simulink model "twsbr_fuzzy_pid"  (R2026a)
settings: Solver=ode45  StopTime=8.0  MaxStep=0.001  RelTol=1e-9  AbsTol=1e-11
model workspace (MAT data in the model file):
  controller_reset_data = [0  1; 0.001  0; 8  0]
  disturbance_force_data = [0  0; 8  0]
  disturbance_torque_data = [0  0; 8  0]
  position_reference_data = [0  0; 8  0]
settings Model: Creator=Linxiuqi  LastModifiedBy=Linxiuqi

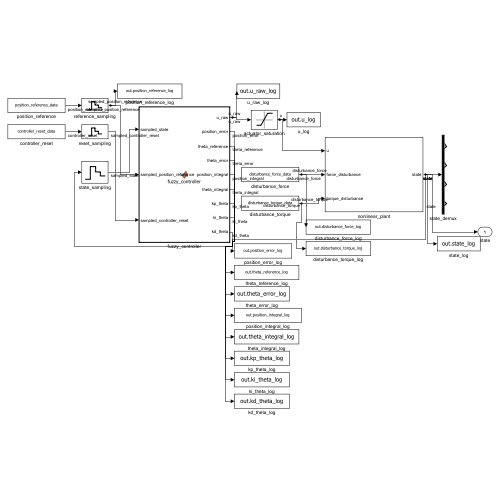
[thumbnail: Simulink's stored preview of the top-level diagram]
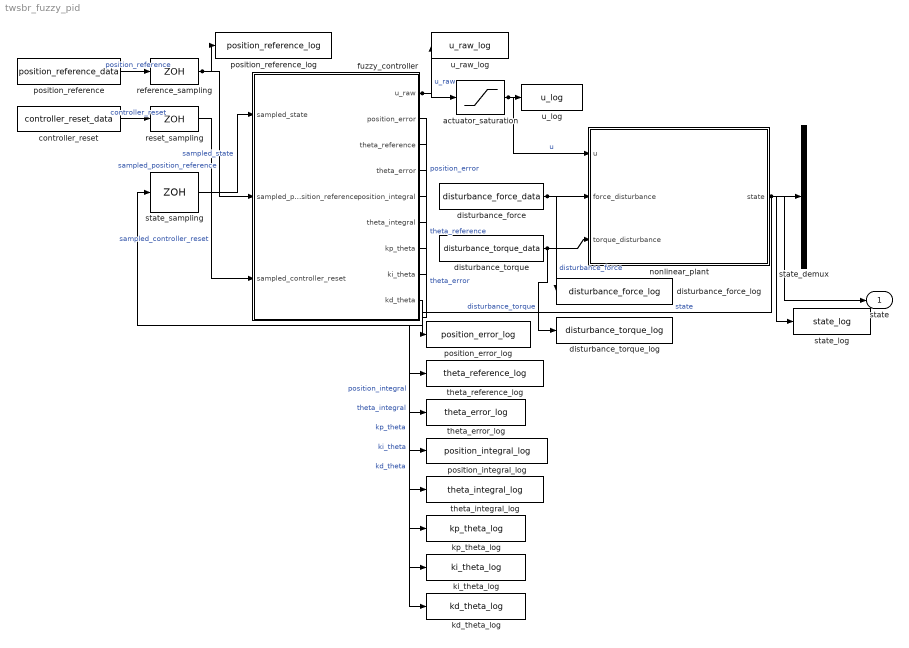
== system twsbr_fuzzy_pid ==
  actuator_saturation : Saturate  UpperLimit=1  LowerLimit=-1
  controller_reset : FromWorkspace  VariableName=controller_reset_data  Interpolate=off  OutputAfterFinalValue=Holding final value
  disturbance_force : FromWorkspace  VariableName=disturbance_force_data  Interpolate=off  OutputAfterFinalValue=Holding final value
  disturbance_force_log : ToWorkspace  VariableName=disturbance_force_log  SaveFormat=Structure With Time  SampleTime=-1
  disturbance_torque : FromWorkspace  VariableName=disturbance_torque_data  Interpolate=off  OutputAfterFinalValue=Holding final value
  disturbance_torque_log : ToWorkspace  VariableName=disturbance_torque_log  SaveFormat=Structure With Time  SampleTime=-1
  fuzzy_controller : MATLAB Function  TreatAsAtomicUnit=on
  kd_theta_log : ToWorkspace  VariableName=kd_theta_log  SaveFormat=Structure With Time  SampleTime=-1
  ki_theta_log : ToWorkspace  VariableName=ki_theta_log  SaveFormat=Structure With Time  SampleTime=-1
  kp_theta_log : ToWorkspace  VariableName=kp_theta_log  SaveFormat=Structure With Time  SampleTime=-1
  nonlinear_plant : Subsystem
  position_error_log : ToWorkspace  VariableName=position_error_log  SaveFormat=Structure With Time  SampleTime=-1
  position_integral_log : ToWorkspace  VariableName=position_integral_log  SaveFormat=Structure With Time  SampleTime=-1
  position_reference : FromWorkspace  VariableName=position_reference_data  Interpolate=off  OutputAfterFinalValue=Holding final value
  position_reference_log : ToWorkspace  VariableName=position_reference_log  SaveFormat=Structure With Time  SampleTime=-1
  reference_sampling : ZeroOrderHold  SampleTime=0.01
  reset_sampling : ZeroOrderHold  SampleTime=0.01
  state_demux : Demux
  state_log : ToWorkspace  VariableName=state_log  SaveFormat=Structure With Time  SampleTime=-1
  state_sampling : ZeroOrderHold  SampleTime=0.01
  theta_error_log : ToWorkspace  VariableName=theta_error_log  SaveFormat=Structure With Time  SampleTime=-1
  theta_integral_log : ToWorkspace  VariableName=theta_integral_log  SaveFormat=Structure With Time  SampleTime=-1
  theta_reference_log : ToWorkspace  VariableName=theta_reference_log  SaveFormat=Structure With Time  SampleTime=-1
  u_log : ToWorkspace  VariableName=u_log  SaveFormat=Structure With Time  SampleTime=-1
  u_raw_log : ToWorkspace  VariableName=u_raw_log  SaveFormat=Structure With Time  SampleTime=-1
  state : Outport
  wires:
  position_reference/1 -> reference_sampling/1  "position_reference"
  reference_sampling/1 -> fuzzy_controller/2(sampled_position_reference), position_reference_log/1  "sampled_position_reference"
  controller_reset/1 -> reset_sampling/1  "controller_reset"
  reset_sampling/1 -> fuzzy_controller/3(sampled_controller_reset)  "sampled_controller_reset"
  nonlinear_plant/1(state) -> state_sampling/1, state_demux/1, state/1, state_log/1  "state"
  state_sampling/1 -> fuzzy_controller/1(sampled_state)  "sampled_state"
  fuzzy_controller/1(u_raw) -> actuator_saturation/1, u_raw_log/1  "u_raw"
  fuzzy_controller/2(position_error) -> position_error_log/1  "position_error"
  fuzzy_controller/3(theta_reference) -> theta_reference_log/1  "theta_reference"
  fuzzy_controller/4(theta_error) -> theta_error_log/1  "theta_error"
  fuzzy_controller/5(position_integral) -> position_integral_log/1  "position_integral"
  fuzzy_controller/6(theta_integral) -> theta_integral_log/1  "theta_integral"
  fuzzy_controller/7(kp_theta) -> kp_theta_log/1  "kp_theta"
  fuzzy_controller/8(ki_theta) -> ki_theta_log/1  "ki_theta"
  fuzzy_controller/9(kd_theta) -> kd_theta_log/1  "kd_theta"
  actuator_saturation/1 -> nonlinear_plant/1(u), u_log/1  "u"
  disturbance_force/1 -> nonlinear_plant/2(force_disturbance), disturbance_force_log/1  "disturbance_force"
  disturbance_torque/1 -> nonlinear_plant/3(torque_disturbance), disturbance_torque_log/1  "disturbance_torque"

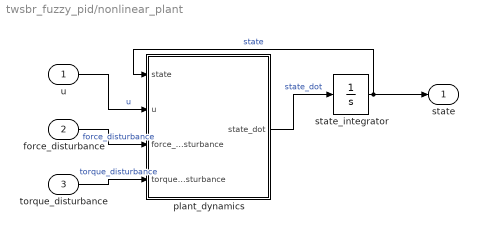
== system twsbr_fuzzy_pid/nonlinear_plant ==
  u : Inport
  force_disturbance : Inport  Port=2
  torque_disturbance : Inport  Port=3
  plant_dynamics : MATLAB Function  TreatAsAtomicUnit=on
  state_integrator : Integrator  InitialCondition=[0;0;0;0]
  state : Outport
  wires:
  plant_dynamics/1(state_dot) -> state_integrator/1  "state_dot"
  torque_disturbance/1 -> plant_dynamics/4(torque_disturbance)  "torque_disturbance"
  force_disturbance/1 -> plant_dynamics/3(force_disturbance)  "force_disturbance"
  u/1 -> plant_dynamics/2(u)  "u"
  state_integrator/1 -> state/1, plant_dynamics/1(state)  "state"

== matlab function twsbr_fuzzy_pid/nonlinear_plant/plant_dynamics ==
  data: state input; u input; state_dot output; force_disturbance input; torque_disturbance input
function state_dot = plant_dynamics(state, u, force_disturbance, torque_disturbance)
%#codegen
body_mass = 1.2;
wheel_mass = 0.29999999999999999;
com_length = 0.17999999999999999;
body_inertia = 0.025000000000000001;
damping = 0.050000000000000003;
gravity = 9.8100000000000005;
motor_gain = 12;
x_dot = state(2);
theta = state(3);
theta_dot = state(4);
force = motor_gain * u + force_disturbance;
mass_sum = wheel_mass + body_mass;
rotational_term = body_inertia + body_mass * com_length^2;
coupling = body_mass * com_length * cos(theta);
rhs_position = force - damping * x_dot + body_mass * com_length * theta_dot^2 * sin(theta);
rhs_angle = body_mass * gravity * com_length * sin(theta) + torque_disturbance;
determinant = mass_sum * rotational_term - coupling^2;
x_ddot = (rotational_term * rhs_position - coupling * rhs_angle) / determinant;
theta_ddot = (-coupling * rhs_position + mass_sum * rhs_angle) / determinant;
state_dot = [x_dot; x_ddot; theta_dot; theta_ddot];
end

== matlab function twsbr_fuzzy_pid/fuzzy_controller ==
  data: sampled_state input; u_raw output; sampled_position_reference input; sampled_controller_reset input; position_error output; theta_reference output; theta_error output; position_integral output; theta_integral output; kp_theta output; ki_theta output; kd_theta output
function [u_raw, position_error, theta_reference, theta_error, position_integral, theta_integral, kp_theta, ki_theta, kd_theta] = fuzzy_controller(sampled_state, sampled_position_reference, sampled_controller_reset)
%#codegen
persistent position_integral_state theta_integral_state
if isempty(position_integral_state) || sampled_controller_reset ~= 0
    position_integral_state = 0.0;
    theta_integral_state = 0.0;
end
kp_x = 0.24099999999999999;
ki_x = 0.00039599999999999987;
kd_x = 0.193;
kp_theta_base = 9.254999999999999;
ki_theta_base = 0.049999999999999989;
kd_theta_base = 1.0109999999999999;
alpha_p = 0.20000000000000001;
alpha_i = 0.20000000000000001;
alpha_d = 0.20000000000000001;
theta_error_normalizer = 0.20943951023931956;
theta_rate_normalizer = 2.0943951023931953;
kp_theta_max = 37.019999999999996;
ki_theta_max = 0.19999999999999996;
kd_theta_max = 4.0439999999999996;
sample_time = 0.01;
theta_reference_limit = 0.20943951023931956;
position_integral_limit = 1000000;
theta_integral_limit = 1000000;
u_max = 1;
x = sampled_state(1);
x_dot = sampled_state(2);
theta = sampled_state(3);
theta_dot = sampled_state(4);
position_integral = position_integral_state;
theta_integral = theta_integral_state;
position_error = sampled_position_reference - x;
theta_reference_raw = kp_x * position_error + ki_x * position_integral - kd_x * x_dot;
theta_reference = min(max(theta_reference_raw, -theta_reference_limit), theta_reference_limit);
theta_error = theta - theta_reference;
[adjustments, ~] = fuzzy_pid_inference(theta_error / theta_error_normalizer, theta_dot / theta_rate_normalizer);
kp_theta = clamp_gain(kp_theta_base * (1.0 + alpha_p * adjustments.delta_kp), kp_theta_max);
ki_theta = clamp_gain(ki_theta_base * (1.0 + alpha_i * adjustments.delta_ki), ki_theta_max);
kd_theta = clamp_gain(kd_theta_base * (1.0 + alpha_d * adjustments.delta_kd), kd_theta_max);
u_raw = kp_theta * theta_error + ki_theta * theta_integral + kd_theta * theta_dot;
position_integral_state = min(max(position_integral + sample_time * position_error, -position_integral_limit), position_integral_limit);
if abs(u_raw) <= u_max || theta_error * u_raw < 0
    theta_integral_state = min(max(theta_integral + sample_time * theta_error, -theta_integral_limit), theta_integral_limit);
end
end
function gain = clamp_gain(value, gain_max)
gain = min(max(value, 0.0), gain_max);
end
